simulink model "Single_Phase_AC_AC_Frequency_Converter"  (Simulink 7.5)
settings: Solver=ode15s  StartTime=0.0  StopTime=1  RelTol=1e-3
libraries: powerlib x14, powerlib_extras x2
settings Model: Creator=lm  LastModifiedBy=lm

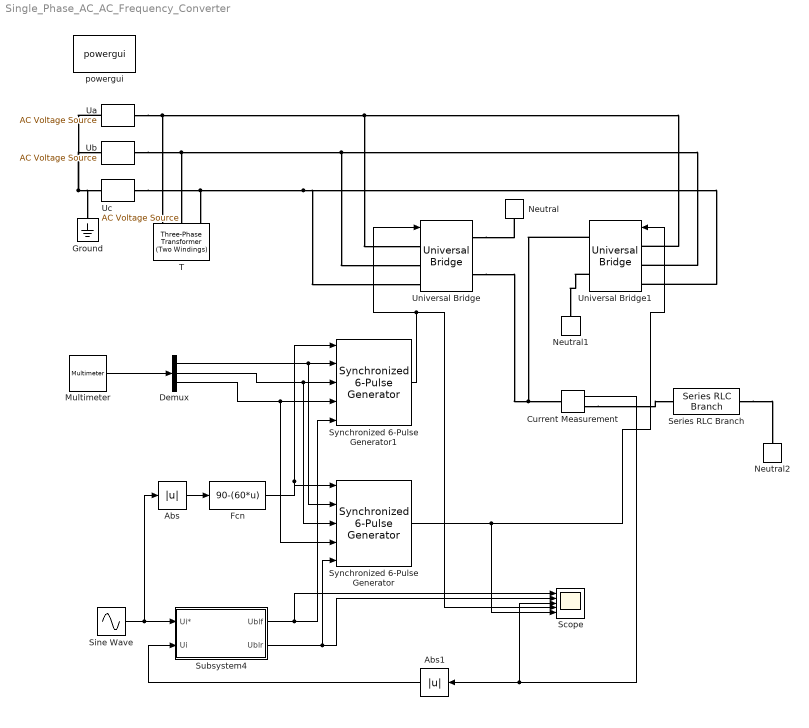
== system Single_Phase_AC_AC_Frequency_Converter ==
  Abs : Abs  OutDataType=fixdt(1, 16)  OutScaling=2^0
  Abs1 : Abs  OutDataType=fixdt(1, 16)  OutScaling=2^0
  Current Measurement : powerlib/Measurements/Current Measurement  DialogController=POWERSYS.PowerSysDialog  SystemSampleTime=-1  PhasorSimulation=off  OutputType=Complex  PSBequivalent=0
  Demux : Demux  Outputs=3
  Fcn : Fcn  Expr=90-(60*u)
  Ground : powerlib/Elements/Ground  DialogController=POWERSYS.PowerSysDialog  PhysicalDomain=powersysdomain  SubClassName=unknown  LeftPortType=p1  RightPortType=p1  LConnTagsString=a
  Multimeter : powerlib/Measurements/Multimeter  SystemSampleTime=-1  PhasorSimulation=off  OutputType=Complex  sel=[9 8 7]  L=9  Gain=[1 1 1]  yselected={'Usrc: Ua','Usrc: Ub','Usrc: Uc'};  PSBOutputType=1  PSBequivalent=0  AxesSetting=[0,0.1,-100,100]  Display=0  SavedBlockNames=-11
  Neutral : powerlib/Elements/Neutral  DialogController=POWERSYS.PowerSysDialog  PhysicalDomain=powersysdomain  SubClassName=unknown  LeftPortType=p1  RightPortType=p1  LConnTagsString=a  NodeNumber=10
  Neutral1 : powerlib/Elements/Neutral  DialogController=POWERSYS.PowerSysDialog  PhysicalDomain=powersysdomain  SubClassName=unknown  LeftPortType=p1  RightPortType=p1  LConnTagsString=a  NodeNumber=10
  Neutral2 : powerlib/Elements/Neutral  DialogController=POWERSYS.PowerSysDialog  PhysicalDomain=powersysdomain  SubClassName=unknown  LeftPortType=p1  RightPortType=p1  LConnTagsString=a  NodeNumber=10
  Scope : Scope  NumInputPorts=5
      settings: YMin=-5~-5~-5~-5~-5  YMax=5~5~5~5~5
  Series RLC Branch : powerlib/Elements/Series RLC Branch  DialogController=POWERSYS.PowerSysDialog  PhysicalDomain=powersysdomain  SubClassName=unknown  LeftPortType=p1  RightPortType=p1  LConnTagsString=__new0  RConnTagsString=__new0  BranchType=RL  Resistance=1  Inductance=1e-3  SetiL0=off  InitialCurrent=0  Capacitance=1e-6  Setx0=off  InitialVoltage=0  Measurements=None
  Sine Wave : Sin  Amplitude=1  Bias=0  Frequency=1  Phase=0  Samples=10  SampleTime=0  Offset=0
  Subsystem4 : Subsystem
  Synchronized 6-Pulse Generator : powerlib_extras/Control  Blocks/Synchronized 6-Pulse Generator  DialogController=POWERSYS.PowerSysDialog  SystemSampleTime=-1  freq=60  pwidth=10  Double_Pulse=off
  Synchronized 6-Pulse Generator1 : powerlib_extras/Control  Blocks/Synchronized 6-Pulse Generator  DialogController=POWERSYS.PowerSysDialog  SystemSampleTime=-1  freq=60  pwidth=10  Double_Pulse=off
  T : powerlib/Elements/Three-Phase Transformer (Two Windings)  DialogController=POWERSYS.PowerSysDialog  SystemSampleTime=-1  Winding1Connection=Yg  UNITS=pu  NominalPower=[ 250e6 , 60 ]  Winding1=[ 735e3 , 0.002 , 0.08 ]  Winding2Connection=Yg  Winding2=[ 315e3 , 0.002 , 0.08 ]  SetSaturation=off  Rm=500  Lm=500  Saturation=[ 0,0 ; 0.0024,1.2 ; 1.0,1.52 ]  Hysteresis=off  DataFile='hysteresis'  SetInitialFlux=off  InitialFluxes=[ 0.8 , -0.8 , 0.7 ]  Measurements=Winding voltages  MoreParameters=off  BreakLoop=off  DataType=off  TransfoNumber=1
  Ua : powerlib/Electrical Sources/AC Voltage Source  DialogController=POWERSYS.PowerSysDialog  SystemSampleTime=-1  Amplitude=220*sqrt(2)  Phase=0  Frequency=50  SampleTime=0  Measurements=Voltage
  Ub : powerlib/Electrical Sources/AC Voltage Source  DialogController=POWERSYS.PowerSysDialog  SystemSampleTime=-1  Amplitude=220*sqrt(2)  Phase=-120  Frequency=50  SampleTime=0  Measurements=Voltage
  Uc : powerlib/Electrical Sources/AC Voltage Source  DialogController=POWERSYS.PowerSysDialog  SystemSampleTime=-1  Amplitude=220*sqrt(2)  Phase=-240  Frequency=50  SampleTime=0  Measurements=Voltage
  Universal Bridge : powerlib/Power Electronics/Universal Bridge  DialogController=POWERSYS.PowerSysDialog  SystemSampleTime=-1  Arms=3  SnubberResistance=1e5  SnubberCapacitance=inf  Device=Thyristors  Ron=1e-3  Lon=0  ForwardVoltages="[  0  0  ]"  ForwardVoltage=0  GTOparameters=[ 10e-6 , 20e-6 ]  IGBTparameters=[ 1e-6 , 2e-6 ]  Measurements=None  Measurements_2=None  converterType=Rectifier
  Universal Bridge1 : powerlib/Power Electronics/Universal Bridge  DialogController=POWERSYS.PowerSysDialog  SystemSampleTime=-1  Arms=3  SnubberResistance=1e5  SnubberCapacitance=inf  Device=Thyristors  Ron=1e-3  Lon=0  ForwardVoltages="[  0  0  ]"  ForwardVoltage=0  GTOparameters=[ 10e-6 , 20e-6 ]  IGBTparameters=[ 1e-6 , 2e-6 ]  Measurements=None  Measurements_2=None  converterType=Rectifier
  powergui : powerlib/powergui  Priority=1  SystemSampleTime=-1  SimulationMode=Continuous  SampleTime=50e-6  frequency=60  SPID=off  DisableSnubberDevices=off  DisableRonSwitches=off  DisableVfSwitches=off  SwTol=0  Interpol=off  frequencyindice=50  echomessages=off  HookPort=off  DisplayEquations=off  FunctionMessages=off  EnableUseOfTLC=off  x0status=blocks  RestoreLinks=warning  ResistiveCurrentMeasurement=off  Ylog=off  Xlog=on  ShowGrid=off  save=off  variable=ZData  ZoomFFT=off  StartTime=0.0  cycles=1  DisplayStyle=1  FreqAxis=off  MaxFrequency=1000  frequencyindicesteady=1  display=off  methode=off
  wires:
  Sine Wave/1 -> Subsystem4/1(Ui*), Abs/1
  Abs/1 -> Fcn/1
  Fcn/1 -> Synchronized 6-Pulse Generator1/1, Synchronized 6-Pulse Generator/1
  Subsystem4/1(Ublf) -> Synchronized 6-Pulse Generator1/5, Scope/1
  Subsystem4/2(Ublr) -> Synchronized 6-Pulse Generator/5, Scope/2
  Synchronized 6-Pulse Generator1/1 -> Universal Bridge/1, Scope/4
  Synchronized 6-Pulse Generator/1 -> Universal Bridge1/1, Scope/5
  Current Measurement/1 -> Abs1/1, Scope/3
  Abs1/1 -> Subsystem4/2(Ui)
  Multimeter/1 -> Demux/1
  Demux/1 -> Synchronized 6-Pulse Generator1/2, Synchronized 6-Pulse Generator/2
  Demux/2 -> Synchronized 6-Pulse Generator1/3, Synchronized 6-Pulse Generator/3
  Demux/3 -> Synchronized 6-Pulse Generator1/4, Synchronized 6-Pulse Generator/4
  connections:
  Ua/LConn1 -- Ub/LConn1 -- Uc/LConn1 -- Ground/LConn1
  Ua/RConn1 -- Universal Bridge1/LConn1 -- Universal Bridge/LConn1 -- T/LConn1
  Ub/RConn1 -- Universal Bridge1/LConn2 -- Universal Bridge/LConn2 -- T/LConn2
  Uc/RConn1 -- Universal Bridge1/LConn3 -- Universal Bridge/LConn3 -- T/LConn3
  Universal Bridge/RConn1 -- Neutral/LConn1
  Universal Bridge1/RConn2 -- Neutral1/LConn1
  Universal Bridge/RConn2 -- Current Measurement/LConn1 -- Universal Bridge1/RConn1
  Current Measurement/RConn1 -- Series RLC Branch/LConn1
  Series RLC Branch/RConn1 -- Neutral2/LConn1

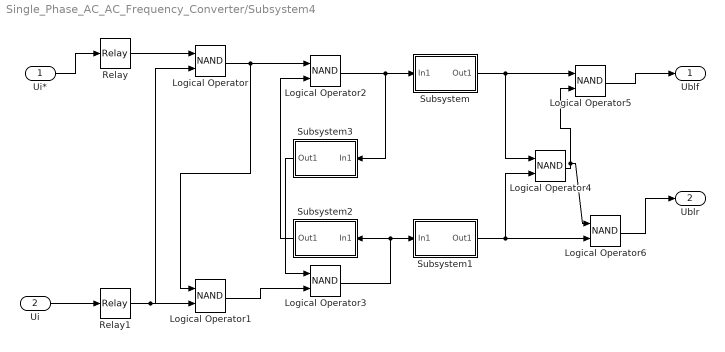
== system Single_Phase_AC_AC_Frequency_Converter/Subsystem4 ==
  Ui* : Inport  OutDataType=fixdt(1, 16)  OutScaling=2^0
  Ui : Inport  Port=2  OutDataType=fixdt(1, 16)  OutScaling=2^0
  Logical Operator : Logic  Operator=NAND  AllPortsSameDT=off  LogicDataType=fixdt(0, 8)
  Logical Operator{1..6} (6 alike) : Logic  Operator=NAND  AllPortsSameDT=off  OutDataTypeMode=boolean  LogicDataType=fixdt(0, 8)  OutDataTypeStr=boolean
  Relay : Relay  OnSwitchValue=0.001  OffSwitchValue=-0.001  OutDataType=fixdt(1, 16)  OutScaling=2^0
  Relay1 : Relay  OnSwitchValue=0.5  OffSwitchValue=0.01  OnOutputValue=0  OffOutputValue=1  OutDataType=fixdt(1, 16)  OutScaling=2^0
  Subsystem : Subsystem
  Subsystem1 : Subsystem
  Subsystem2 : Subsystem
  Subsystem3 : Subsystem
  Ublf : Outport  OutDataType=fixdt(1, 16)  OutScaling=2^0
  Ublr : Outport  Port=2  OutDataType=fixdt(1, 16)  OutScaling=2^0
  wires:
  Relay/1 -> Logical Operator/1
  Relay1/1 -> Logical Operator/2, Logical Operator1/2
  Logical Operator/1 -> Logical Operator2/1, Logical Operator1/1
  Subsystem2/1(Out1) -> Logical Operator2/2
  Subsystem3/1(Out1) -> Logical Operator3/1
  Logical Operator1/1 -> Logical Operator3/2
  Logical Operator3/1 -> Subsystem2/1(In1), Subsystem1/1(In1)
  Logical Operator2/1 -> Subsystem3/1(In1), Subsystem/1(In1)
  Subsystem/1(Out1) -> Logical Operator4/1, Logical Operator5/1
  Subsystem1/1(Out1) -> Logical Operator4/2, Logical Operator6/2
  Logical Operator4/1 -> Logical Operator5/2, Logical Operator6/1
  Logical Operator5/1 -> Ublf/1
  Logical Operator6/1 -> Ublr/1
  Ui*/1 -> Relay/1
  Ui/1 -> Relay1/1

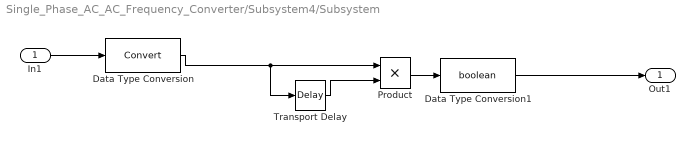
== system Single_Phase_AC_AC_Frequency_Converter/Subsystem4/Subsystem ==
  In1 : Inport  OutDataType=fixdt(1, 16)  OutScaling=2^0
  Data Type Conversion : DataTypeConversion  OutDataType=fixdt(1, 16)  OutScaling=2^0
  Data Type Conversion1 : DataTypeConversion  OutDataTypeMode=boolean  OutDataType=fixdt(1, 16)  OutScaling=2^0  OutDataTypeStr=boolean
  Product : Product  OutDataType=fixdt(1, 16)  OutScaling=2^0  RndMeth=Zero
  Transport Delay : TransportDelay  DelayTime=7e-3
  Out1 : Outport  OutDataType=fixdt(1, 16)  OutScaling=2^0
  wires:
  Data Type Conversion1/1 -> Out1/1
  Product/1 -> Data Type Conversion1/1
  In1/1 -> Data Type Conversion/1
  Data Type Conversion/1 -> Product/1, Transport Delay/1
  Transport Delay/1 -> Product/2

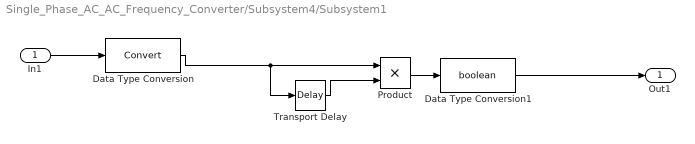
== system Single_Phase_AC_AC_Frequency_Converter/Subsystem4/Subsystem1 ==
  In1 : Inport  OutDataType=fixdt(1, 16)  OutScaling=2^0
  Data Type Conversion : DataTypeConversion  OutDataType=fixdt(1, 16)  OutScaling=2^0
  Data Type Conversion1 : DataTypeConversion  OutDataTypeMode=boolean  OutDataType=fixdt(1, 16)  OutScaling=2^0  OutDataTypeStr=boolean
  Product : Product  OutDataType=fixdt(1, 16)  OutScaling=2^0  RndMeth=Zero
  Transport Delay : TransportDelay  DelayTime=7e-3
  Out1 : Outport  OutDataType=fixdt(1, 16)  OutScaling=2^0
  wires:
  Transport Delay/1 -> Product/2
  Data Type Conversion/1 -> Transport Delay/1, Product/1
  In1/1 -> Data Type Conversion/1
  Product/1 -> Data Type Conversion1/1
  Data Type Conversion1/1 -> Out1/1

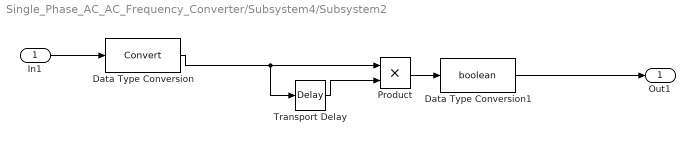
== system Single_Phase_AC_AC_Frequency_Converter/Subsystem4/Subsystem2 ==
  In1 : Inport  OutDataType=fixdt(1, 16)  OutScaling=2^0
  Data Type Conversion : DataTypeConversion  OutDataType=fixdt(1, 16)  OutScaling=2^0
  Data Type Conversion1 : DataTypeConversion  OutDataTypeMode=boolean  OutDataType=fixdt(1, 16)  OutScaling=2^0  OutDataTypeStr=boolean
  Product : Product  OutDataType=fixdt(1, 16)  OutScaling=2^0  RndMeth=Zero
  Transport Delay : TransportDelay  DelayTime=3e-3
  Out1 : Outport  OutDataType=fixdt(1, 16)  OutScaling=2^0
  wires:
  Data Type Conversion1/1 -> Out1/1
  Product/1 -> Data Type Conversion1/1
  In1/1 -> Data Type Conversion/1
  Data Type Conversion/1 -> Product/1, Transport Delay/1
  Transport Delay/1 -> Product/2

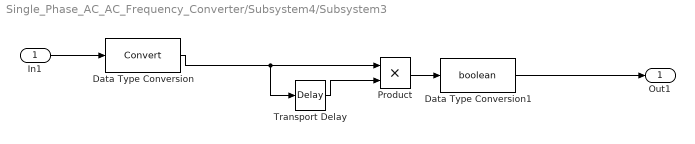
== system Single_Phase_AC_AC_Frequency_Converter/Subsystem4/Subsystem3 ==
  In1 : Inport  OutDataType=fixdt(1, 16)  OutScaling=2^0
  Data Type Conversion : DataTypeConversion  OutDataType=fixdt(1, 16)  OutScaling=2^0
  Data Type Conversion1 : DataTypeConversion  OutDataTypeMode=boolean  OutDataType=fixdt(1, 16)  OutScaling=2^0  OutDataTypeStr=boolean
  Product : Product  OutDataType=fixdt(1, 16)  OutScaling=2^0  RndMeth=Zero
  Transport Delay : TransportDelay  DelayTime=3e-3
  Out1 : Outport  OutDataType=fixdt(1, 16)  OutScaling=2^0
  wires:
  Transport Delay/1 -> Product/2
  Data Type Conversion/1 -> Transport Delay/1, Product/1
  In1/1 -> Data Type Conversion/1
  Product/1 -> Data Type Conversion1/1
  Data Type Conversion1/1 -> Out1/1
